simulink model "idex3_guangyi"  (R2019b)
settings: Solver=ode45  StartTime=0.0  StopTime=800  RelTol=1e-3  EnableMultiTasking=on
libraries: simulink_extras x5, simulink x1
settings Model: Creator=erange  LastModifiedBy=erange
settings DataIOCC: LimitDataPoints=on  SaveFormat=Array  SignalLoggingSaveFormat=ModelDataLogs  ReturnWorkspaceOutputs=off  SignalLoggingName=sigsOut
settings DebuggingCC: SaveWithParameterizedLinksMsg=none  UnderspecifiedInitializationDetection=Classic  MergeDetectMultiDrivingBlocksExec=none  SignalResolutionControl=TryResolveAllWithWarning  MultiTaskDSMMsg=warning  MultiTaskCondExecSysMsg=none
settings HardwareCC: ProdBitPerPointer=32  ProdBitPerSizeT=32  ProdBitPerPtrDiffT=32  ProdLargestAtomicFloat=None  ProdIntDivRoundTo=Undefined  ProdEndianess=Unspecified  ProdWordSize=32  ProdHWDeviceType=32-bit Generic  TargetUnknown=on
settings ModelReferenceCC: PropagateSignalLabelsOutOfModel=off
settings GRTTargetCC: CombineOutputUpdateFcns=off  GRTInterface=on
settings ConfigComp: CovMetricSettings=dw  CovHtmlReporting=on  CovSaveCumulativeToWorkspaceVar=on  CovSaveSingleToWorkspaceVar=on

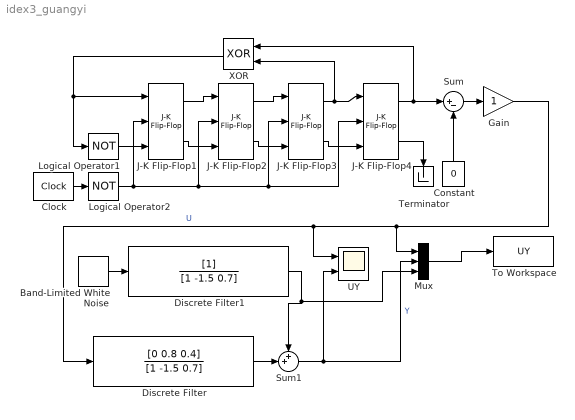
== system idex3_guangyi ==
  Band-Limited White Noise : simulink/Sources/Band-Limited White Noise  Cov=0.15  Ts=1  seed=[23341]
  Clock : simulink_extras/Flip Flops/Clock  period=1
  Constant : Constant  Value=0
  Discrete Filter : DiscreteFilter  Numerator=[0 0.8 0.4]  Denominator=[1 -1.5 0.7]  SampleTime=1
  Discrete Filter1 : DiscreteFilter  Denominator=[1 -1.5 0.7]  SampleTime=1
  Gain : Gain  SaturateOnIntegerOverflow=on  OutDataTypeStr=Inherit: Same as input  ParamDataTypeStr=Inherit: Same as input
  J-K Flip-Flop{1..4} (4 alike) : simulink_extras/Flip Flops/J-K Flip-Flop  initial_condition=1
      settings: SourceProductName=Simulink
  Logical Operator1 : Logic  Operator=NOT  Inputs=1  AllPortsSameDT=off
  Logical Operator2 : Logic  Operator=NOT  Inputs=1  AllPortsSameDT=off
  Mux : Mux  Inputs=3
  Sum : Sum  Inputs=|+-  SaturateOnIntegerOverflow=on
  Sum1 : Sum  Inputs=++|  SaturateOnIntegerOverflow=on
  Terminator : Terminator
  To Workspace : ToWorkspace  VariableName=UY  SampleTime=1
  UY : Scope  NumInputPorts=2
  XOR : Logic  Operator=XOR  AllPortsSameDT=off
  wires:
  J-K Flip-Flop1/1 -> J-K Flip-Flop2/1
  J-K Flip-Flop4/1 -> XOR/1, Sum/1
  XOR/1 -> J-K Flip-Flop1/1, Logical Operator1/1
  J-K Flip-Flop3/2 -> J-K Flip-Flop4/3
  J-K Flip-Flop1/2 -> J-K Flip-Flop2/3
  Logical Operator1/1 -> J-K Flip-Flop1/3
  J-K Flip-Flop3/1 -> XOR/2, J-K Flip-Flop4/1
  J-K Flip-Flop4/2 -> Terminator/1
  Sum/1 -> Gain/1
  Constant/1 -> Sum/2
  J-K Flip-Flop2/2 -> J-K Flip-Flop3/3
  J-K Flip-Flop2/1 -> J-K Flip-Flop3/1
  Gain/1 -> Mux/1, Discrete Filter/1, UY/1  "U"
  Mux/1 -> To Workspace/1
  Clock/1 -> Logical Operator2/1
  Logical Operator2/1 -> J-K Flip-Flop4/2, J-K Flip-Flop3/2, J-K Flip-Flop2/2, J-K Flip-Flop1/2
  Discrete Filter/1 -> Sum1/2
  Sum1/1 -> Mux/2, UY/2  "Y"
  Discrete Filter1/1 -> Mux/3, Sum1/1
  Band-Limited White Noise/1 -> Discrete Filter1/1
